simulink model "RR"  (R2024a)
settings: Solver=VariableStepAuto  StartTime=0.0  StopTime=15  RelTol=1e-3  EnableMultiTasking=on
libraries: sm_lib x12, nesl_utility x7
settings Model: Creator=Shashank  LastModifiedBy=ASUS
settings SolverCC: AlgebraicLoopSolver=TrustRegion
settings DataIOCC: LimitDataPoints=on
settings OptimizationCC: LifeSpan=inf
settings DebuggingCC: UnconnectedInputMsg=warning  UnconnectedOutputMsg=warning  UnconnectedLineMsg=warning  AllowSymbolicDim=off  SFUnexpectedBacktrackingDiag=warning  SFNoUnconditionalDefaultTransitionDiag=warning  SFExecutionAtInitializationDiag=none  ArithmeticOperatorsInVariantConditions=warning
settings ModelReferenceCC: EnableRefExpFcnMdlSchedulingChecks=on
settings SFSimCC: SimUseLocalCustomCode=off  CustomCodeUndefinedFunction=UseInterfaceOnly
settings RTWCC: RTWUseLocalCustomCode=off  GPUComputeCapability=3.5
settings CodeAppCC: StateflowObjectComments=on
settings GRTTargetCC: TargetLangStandard=C89/C90 (ANSI)
settings ConfigComp: CovMetricSettings=dw  CovSaveCumulativeToWorkspaceVar=on  CovSaveSingleToWorkspaceVar=on  CovExternalEMLEnable=off  CovSFcnEnable=off
settings SimscapeCC: SimscapeNominalValues="[{\"value\":\"10\",\"unit\":\"V\"},{\"value\":\"1\",\"unit\":\"A\"},{\"value\":\"10\",\"unit\":\"N*m\"},{\"value\":\"10\",\"unit\":\"bar\"},{\"value\":\"100\",\"unit\":\"kJ/kg\"},{\"value\":\"1\",\"unit\":\"kW\"},{\"value\":\"300\",\"unit\":\"K\"},{\"value\":\"100\",\"unit\":\"cm^3/s\"},{\"value\":\"1\",\"unit\":\"kN\"},{\"value\":\"1\",\"unit\":\"g/cm^3\"},{\"value\":\"1\",\"unit\":\"l\"},{\"value\":\"1\",\"unit\":\"cm^2\"},{\"value\":\"60\",\"unit\":\"Hz\"}]"  SimscapeLogType=all  SimscapeLogDataHistory=10000
settings ConfigurationSet: Description=SimMechanics 2G

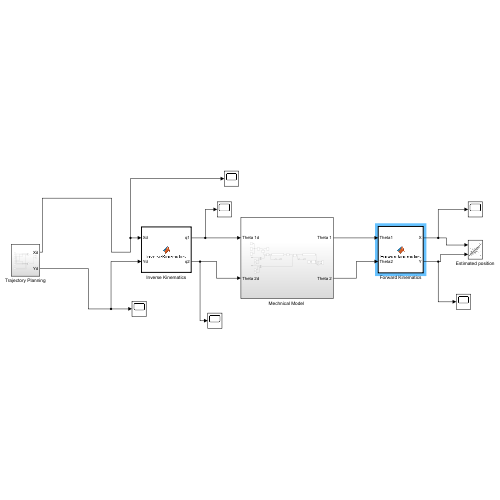
[thumbnail: Simulink's stored preview of the top-level diagram]
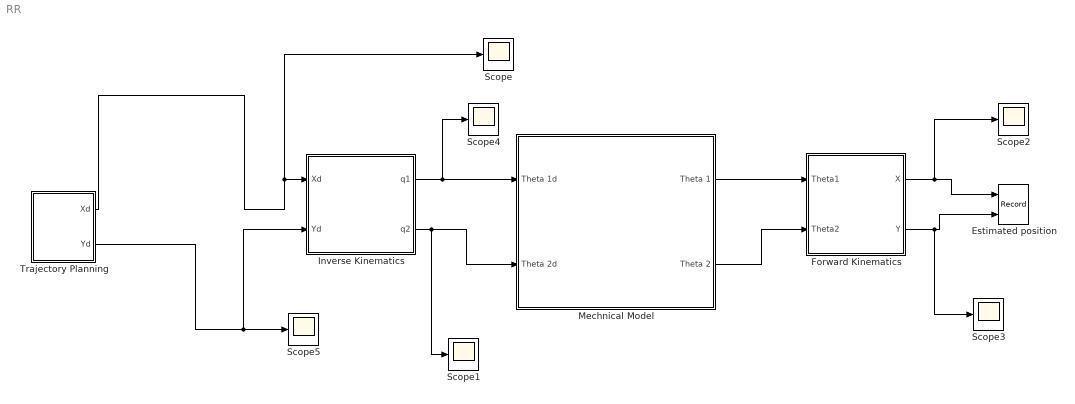
== system RR ==
  Estimated position : Record  FileSettingsInternal="{\"entries\":[{\"content\":{\"excelSettings\":{\"content\":{},\"type\":\"Streamout.ExcelSettings\"}},\"type\":\"Streamout.FileSettingStorage\",\"uuid\":\"\"}],\"packageUris\":[\"http:\\/\\/schema.mathworks.com\\/mf0\\/streamout_blocks\\/R2020a\"],\"version\":\"1.0\"}"  Layout=[1 1]  SignalsInternal="{\"entries\":[{\"content\":{\"signals\":[{\"content\":{\"blockPath\":[],\"dimensions\":[1],\"domain\":\"\",\"lineColor\":\"#a2142f\",\"plots\":[ 1 ],\"port\":1,\"sid\":[\"\"],\"signalID\":1,\"signalName\":\"Forward Kinematics:1\"},\"type\":\"RecordBlkView.Signal\",\"uuid\":\"\"},{\"content\":{\"blockPath\":[],\"dimensions\":[1],\"domain\":\"\",\"lineColor\":\"#139fff\",\"plots\":[ 1 ],\"port\":2,\"sid\":[\"\"],\"signalID\":2,\"signalName\":\"Forward Kinematics:2\"},\"type\":\"RecordBlkView.Signal\",\"uuid\":\"\"}]},\"type\":\"RecordBlkView.InputSignals\",\"uuid\":\"\"}],\"packageUris\":[\"http:\\/\\/schema.mathworks.com\\/mf0\\/streamout_blocks\\/R2020a\"],\"version\":\"1.0\"}"  VisualizationBindings="{\"xyplotplugin\":{\"info\":[{\"series\":[{\"bindingParametersList\":[{\"parameter\":\"X-Axis\",\"signalID\":1,\"signalName\":\"Forward Kinematics:1\"},{\"parameter\":\"Y-Axis\",\"signalID\":2,\"signalName\":\"Forward Kinematics:2\"}],\"seriesID\":0}],\"subplotID\":1}]}}"  CompatibilityTag=XY  st=-1
  Forward Kinematics : MATLAB Function  TreatAsAtomicUnit=on
  Inverse Kinematics : MATLAB Function  TreatAsAtomicUnit=on
  "Mechnical Model " : Subsystem
  Scope{,1..5} (6 alike) : Scope
  Trajectory Planning : Subsystem
  wires:
  Inverse Kinematics/2(q2) -> "Mechnical Model "/2(Theta 2d), Scope1/1
  "Mechnical Model "/1(Theta 1) -> Forward Kinematics/1(Theta1)
  "Mechnical Model "/2(Theta 2) -> Forward Kinematics/2(Theta2)
  Forward Kinematics/1(X) -> Scope2/1, Estimated position/1
  Forward Kinematics/2(Y) -> Scope3/1, Estimated position/2
  Trajectory Planning/1(Xd) -> Inverse Kinematics/1(Xd), Scope/1
  Inverse Kinematics/1(q1) -> Scope4/1, "Mechnical Model "/1(Theta 1d)
  Trajectory Planning/2(Yd) -> Inverse Kinematics/2(Yd), Scope5/1

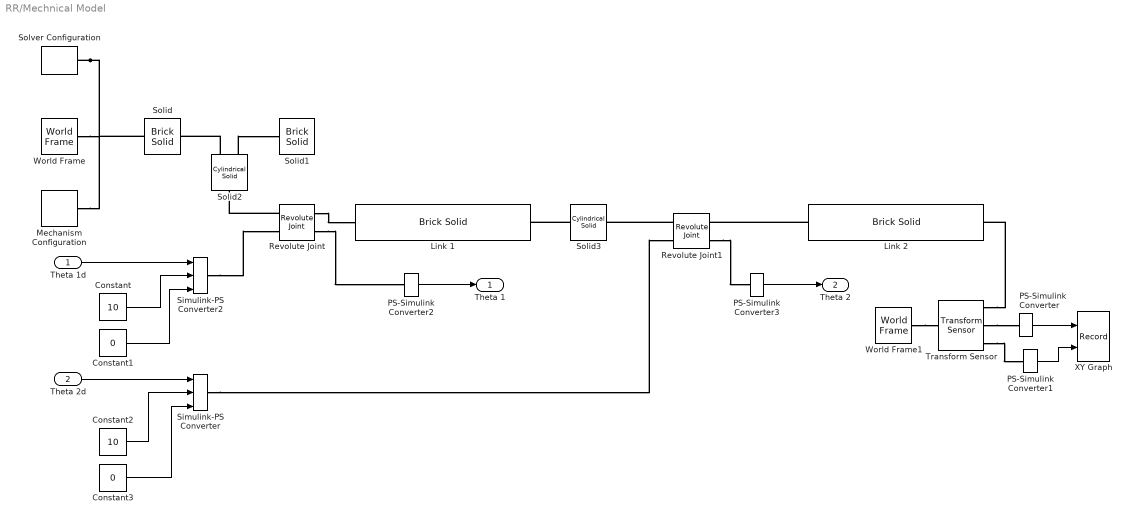
== system RR/Mechnical Model  ==
  Theta 1d : Inport
  Theta 2d : Inport  Port=2
  Constant : Constant  Value=10
  Constant1 : Constant  Value=0
  Constant2 : Constant  Value=10
  Constant3 : Constant  Value=0
  Link 1 : sm_lib/Body Elements/Brick Solid  BrickDimensions=[100 15 5]  BrickDimensionsUnits=cm  ExportEntireGeometry=off  InertiaType=CalculateFromGeometry  BasedOnType=Density  Density=1000  DensityUnits=kg/m^3  Mass=1  MassUnits=kg  CenterOfMass=[0 0 0]  CenterOfMassUnits=m  MomentsOfInertia=[1 1 1]  MomentsOfInertiaUnits=kg*m^2  ProductsOfInertia=[0 0 0]  ProductsOfInertiaUnits=kg*m^2  GraphicType=FromGeometry  MarkerShape=Sphere  MarkerSize=10  GraphicVisPropType=SimpleVisualProperties  GraphicDiffuseColor=[1.0 0.4 0.4]  GraphicOpacity=1.0  GraphicSpecularColor=[0.5 0.5 0.5 1.0]  GraphicAmbientColor=[0.15 0.15 0.15 1.0]  GraphicEmissiveColor=[0.0 0.0 0.0 1.0]  GraphicShininess=75  DoExposeReferenceFrame=off  SerializedFrames=<Frames><Frame><Id>Frame1</Id><Value><Name>L</Name><Origin><Source>GeometricFeature</Source><FeatureName>-x surface</FeatureName></Origin><PrimaryAxis><DefinedDirection>+Z</DefinedDirection><Source>ReferenceFrame</Source><SourceDirection>+Z</SourceDirection><FeatureName></FeatureName></PrimaryAxis><SecondaryAxis><DefinedDirection>+X</DefinedDirection><Source>ReferenceFrame</Source><SourceDirection>+X</SourceDirection><FeatureName></FeatureName></SecondaryAxis></Value></Frame><Frame><Id>Frame2</Id><Value><Name>R</Name><Origin><Source>GeometricFeature</Source><FeatureName>+x surface</FeatureName></Origin><PrimaryAxis><DefinedDirection>+Z</DefinedDirection><Source>ReferenceFrame</Source><SourceDirection>+Z</SourceDirection><FeatureName></FeatureName></PrimaryAxis><SecondaryAxis><DefinedDirection>+X</DefinedDirection><Source>ReferenceFrame</Source><SourceDirection>+X</SourceDirection><FeatureName></FeatureName></SecondaryAxis></Value></Frame></Frames>
  Link 2 : sm_lib/Body Elements/Brick Solid  BrickDimensions=[100 15 5]  BrickDimensionsUnits=cm  ExportEntireGeometry=off  InertiaType=CalculateFromGeometry  BasedOnType=Density  Density=1000  DensityUnits=kg/m^3  Mass=1  MassUnits=kg  CenterOfMass=[0 0 0]  CenterOfMassUnits=m  MomentsOfInertia=[1 1 1]  MomentsOfInertiaUnits=kg*m^2  ProductsOfInertia=[0 0 0]  ProductsOfInertiaUnits=kg*m^2  GraphicType=FromGeometry  MarkerShape=Sphere  MarkerSize=10  GraphicVisPropType=SimpleVisualProperties  GraphicDiffuseColor=[0.0 0.4 0.0]  GraphicOpacity=1.0  GraphicSpecularColor=[0.5 0.5 0.5 1.0]  GraphicAmbientColor=[0.15 0.15 0.15 1.0]  GraphicEmissiveColor=[0.0 0.0 0.0 1.0]  GraphicShininess=75  DoExposeReferenceFrame=off  SerializedFrames=<Frames><Frame><Id>Frame1</Id><Value><Name>L</Name><Origin><Source>GeometricFeature</Source><FeatureName>-x surface</FeatureName></Origin><PrimaryAxis><DefinedDirection>+Z</DefinedDirection><Source>ReferenceFrame</Source><SourceDirection>+Z</SourceDirection><FeatureName></FeatureName></PrimaryAxis><SecondaryAxis><DefinedDirection>+X</DefinedDirection><Source>ReferenceFrame</Source><SourceDirection>+X</SourceDirection><FeatureName></FeatureName></SecondaryAxis></Value></Frame><Frame><Id>Frame2</Id><Value><Name>R</Name><Origin><Source>GeometricFeature</Source><FeatureName>+x surface</FeatureName></Origin><PrimaryAxis><DefinedDirection>+Z</DefinedDirection><Source>ReferenceFrame</Source><SourceDirection>+Z</SourceDirection><FeatureName></FeatureName></PrimaryAxis><SecondaryAxis><DefinedDirection>+X</DefinedDirection><Source>ReferenceFrame</Source><SourceDirection>+X</SourceDirection><FeatureName></FeatureName></SecondaryAxis></Value></Frame></Frames>
  Mechanism Configuration : sm_lib/Utilities/Mechanism Configuration  UniformGravity=Constant  GravityVector=[0 -9.80665 0]  GravityVectorUnits=m/s^2  LinearizationDelta=0.001  JointModeTransitionNonlinearIterations=2
  PS-Simulink Converter{,1..3} (4 alike) : nesl_utility/PS-Simulink Converter  PhysicalDomain=network_engine_domain  SubClassName=ps_output  LeftPortType=input  RightPortType=output  PseudoPeriodic=off  Frequencies=[]  VectorFormat=1-D array  Unit=1  AffineConversion=off
  Revolute Joint : sm_lib/Joints/Revolute Joint  JointMode=Normal  CompositeWrenchDir=FollowerOnBase  CompositeWrenchFrame=BaseFrame  SenseConstraintForce=off  SenseConstraintTorque=off  SenseTotalForce=off  SenseTotalTorque=off  PositionTargetSpecify=off  PositionTargetPriority=High  PositionTargetValue=0  PositionTargetValueUnits=deg  VelocityTargetSpecify=off  VelocityTargetPriority=High  VelocityTargetValue=0  VelocityTargetValueUnits=deg/s  EquilibriumPosition=0  EquilibriumPositionUnits=deg  SpringStiffness=0  SpringStiffnessUnits=N*m/deg  DampingCoefficient=0  DampingCoefficientUnits=N*m/(deg/s)  LowerLimitSpecify=off  LowerLimitBound=-90  LowerLimitBoundUnits=deg  LowerLimitStiffness=1e4  LowerLimitStiffnessUnits=N*m/deg  LowerLimitDamping=10  LowerLimitDampingUnits=N*m/(deg/s)  LowerLimitTransitionRegionWidth=0.1  LowerLimitTransitionRegionWidthUnits=deg  UpperLimitSpecify=off  UpperLimitBound=90  UpperLimitBoundUnits=deg  UpperLimitStiffness=1e4  UpperLimitStiffnessUnits=N*m/deg  UpperLimitDamping=10  UpperLimitDampingUnits=N*m/(deg/s)  UpperLimitTransitionRegionWidth=0.1  UpperLimitTransitionRegionWidthUnits=deg  TorqueActuationMode=ComputedTorque  MotionActuationMode=InputMotion  SensePosition=on  SenseVelocity=off  SenseAcceleration=off  SenseTorqueForce=off  SenseLowerLimitTorqueForce=off  SenseUpperLimitTorqueForce=off
  Revolute Joint1 : sm_lib/Joints/Revolute Joint  JointMode=Normal  CompositeWrenchDir=FollowerOnBase  CompositeWrenchFrame=BaseFrame  SenseConstraintForce=off  SenseConstraintTorque=off  SenseTotalForce=off  SenseTotalTorque=off  PositionTargetSpecify=off  PositionTargetPriority=High  PositionTargetValue=0  PositionTargetValueUnits=deg  VelocityTargetSpecify=off  VelocityTargetPriority=High  VelocityTargetValue=0  VelocityTargetValueUnits=deg/s  EquilibriumPosition=0  EquilibriumPositionUnits=deg  SpringStiffness=0  SpringStiffnessUnits=N*m/deg  DampingCoefficient=0  DampingCoefficientUnits=N*m/(deg/s)  LowerLimitSpecify=off  LowerLimitBound=-90  LowerLimitBoundUnits=deg  LowerLimitStiffness=1e4  LowerLimitStiffnessUnits=N*m/deg  LowerLimitDamping=10  LowerLimitDampingUnits=N*m/(deg/s)  LowerLimitTransitionRegionWidth=0.1  LowerLimitTransitionRegionWidthUnits=deg  UpperLimitSpecify=off  UpperLimitBound=90  UpperLimitBoundUnits=deg  UpperLimitStiffness=1e4  UpperLimitStiffnessUnits=N*m/deg  UpperLimitDamping=10  UpperLimitDampingUnits=N*m/(deg/s)  UpperLimitTransitionRegionWidth=0.1  UpperLimitTransitionRegionWidthUnits=deg  TorqueActuationMode=ComputedTorque  MotionActuationMode=InputMotion  SensePosition=on  SenseVelocity=off  SenseAcceleration=off  SenseTorqueForce=off  SenseLowerLimitTorqueForce=off  SenseUpperLimitTorqueForce=off
  Simulink-PS Converter : nesl_utility/Simulink-PS Converter  PhysicalDomain=network_engine_domain  SubClassName=ps_input  LeftPortType=input  RightPortType=output  PseudoPeriodic=off  Frequencies=[]  NoiseDistribution=none  NoiseParameters=[]  Unit=1  AffineConversion=off  FilteringAndDerivatives=provide  SimscapeFilterOrder=1  InputFilterTimeConstant=0.001  UdotUserProvided=2
  Simulink-PS Converter2 : nesl_utility/Simulink-PS Converter  PhysicalDomain=network_engine_domain  SubClassName=ps_input  LeftPortType=input  RightPortType=output  PseudoPeriodic=off  Frequencies=[]  NoiseDistribution=none  NoiseParameters=[]  Unit=1  AffineConversion=off  FilteringAndDerivatives=provide  SimscapeFilterOrder=1  InputFilterTimeConstant=0.001  UdotUserProvided=2
  Solid : sm_lib/Body Elements/Brick Solid  BrickDimensions=[15 15 5]  BrickDimensionsUnits=cm  ExportEntireGeometry=off  InertiaType=CalculateFromGeometry  BasedOnType=Density  Density=1000  DensityUnits=kg/m^3  Mass=1  MassUnits=kg  CenterOfMass=[0 0 0]  CenterOfMassUnits=m  MomentsOfInertia=[1 1 1]  MomentsOfInertiaUnits=kg*m^2  ProductsOfInertia=[0 0 0]  ProductsOfInertiaUnits=kg*m^2  GraphicType=FromGeometry  MarkerShape=Sphere  MarkerSize=10  GraphicVisPropType=SimpleVisualProperties  GraphicDiffuseColor=[0.0 0.0 0.6]  GraphicOpacity=1.0  GraphicSpecularColor=[0.5 0.5 0.5 1.0]  GraphicAmbientColor=[0.15 0.15 0.15 1.0]  GraphicEmissiveColor=[0.0 0.0 0.0 1.0]  GraphicShininess=75  DoExposeReferenceFrame=on  SerializedFrames=<Frames><Frame><Id>Frame1</Id><Value><Name>F</Name><Origin><Source>GeometricFeature</Source><FeatureName>-z surface</FeatureName></Origin><PrimaryAxis><DefinedDirection>+Z</DefinedDirection><Source>ReferenceFrame</Source><SourceDirection>+Z</SourceDirection><FeatureName></FeatureName></PrimaryAxis><SecondaryAxis><DefinedDirection>+X</DefinedDirection><Source>ReferenceFrame</Source><SourceDirection>+X</SourceDirection><FeatureName></FeatureName></SecondaryAxis></Value></Frame></Frames>
  Solid1 : sm_lib/Body Elements/Brick Solid  BrickDimensions=[15 15 5]  BrickDimensionsUnits=cm  ExportEntireGeometry=off  InertiaType=CalculateFromGeometry  BasedOnType=Density  Density=1000  DensityUnits=kg/m^3  Mass=1  MassUnits=kg  CenterOfMass=[0 0 0]  CenterOfMassUnits=m  MomentsOfInertia=[1 1 1]  MomentsOfInertiaUnits=kg*m^2  ProductsOfInertia=[0 0 0]  ProductsOfInertiaUnits=kg*m^2  GraphicType=FromGeometry  MarkerShape=Sphere  MarkerSize=10  GraphicVisPropType=SimpleVisualProperties  GraphicDiffuseColor=[0.0 0.0 0.6]  GraphicOpacity=1.0  GraphicSpecularColor=[0.5 0.5 0.5 1.0]  GraphicAmbientColor=[0.15 0.15 0.15 1.0]  GraphicEmissiveColor=[0.0 0.0 0.0 1.0]  GraphicShininess=75  DoExposeReferenceFrame=off  SerializedFrames=<Frames><Frame><Id>Frame1</Id><Value><Name>F</Name><Origin><Source>GeometricFeature</Source><FeatureName>+z surface</FeatureName></Origin><PrimaryAxis><DefinedDirection>+Z</DefinedDirection><Source>ReferenceFrame</Source><SourceDirection>+Z</SourceDirection><FeatureName></FeatureName></PrimaryAxis><SecondaryAxis><DefinedDirection>+X</DefinedDirection><Source>ReferenceFrame</Source><SourceDirection>+X</SourceDirection><FeatureName></FeatureName></SecondaryAxis></Value></Frame></Frames>
  Solid2 : sm_lib/Body Elements/Cylindrical Solid  CylinderRadius=5  CylinderRadiusUnits=cm  CylinderLength=6  CylinderLengthUnits=cm  ExportEntireGeometry=off  InertiaType=CalculateFromGeometry  BasedOnType=Density  Density=1000  DensityUnits=kg/m^3  Mass=1  MassUnits=kg  CenterOfMass=[0 0 0]  CenterOfMassUnits=m  MomentsOfInertia=[1 1 1]  MomentsOfInertiaUnits=kg*m^2  ProductsOfInertia=[0 0 0]  ProductsOfInertiaUnits=kg*m^2  GraphicType=FromGeometry  MarkerShape=Sphere  MarkerSize=10  GraphicVisPropType=SimpleVisualProperties  GraphicDiffuseColor=[0.0 0.0 0.6]  GraphicOpacity=1.0  GraphicSpecularColor=[0.5 0.5 0.5 1.0]  GraphicAmbientColor=[0.15 0.15 0.15 1.0]  GraphicEmissiveColor=[0.0 0.0 0.0 1.0]  GraphicShininess=75  DoExposeReferenceFrame=on  SerializedFrames=<Frames><Frame><Id>Frame1</Id><Value><Name>L</Name><Origin><Source>GeometricFeature</Source><FeatureName>top surface</FeatureName></Origin><PrimaryAxis><DefinedDirection>+Z</DefinedDirection><Source>ReferenceFrame</Source><SourceDirection>+Z</SourceDirection><FeatureName></FeatureName></PrimaryAxis><SecondaryAxis><DefinedDirection>+X</DefinedDirection><Source>ReferenceFrame</Source><SourceDirection>+X</SourceDirection><FeatureName></FeatureName></SecondaryAxis></Value></Frame><Frame><Id>Frame2</Id><Value><Name>R</Name><Origin><Source>GeometricFeature</Source><FeatureName>bottom surface</FeatureName></Origin><PrimaryAxis><DefinedDirection>+Z</DefinedDirection><Source>ReferenceFrame</Source><SourceDirection>+Z</SourceDirection><FeatureName></FeatureName></PrimaryAxis><SecondaryAxis><DefinedDirection>+X</DefinedDirection><Source>ReferenceFrame</Source><SourceDirection>+X</SourceDirection><FeatureName></FeatureName></SecondaryAxis></Value></Frame></Frames>
  Solid3 : sm_lib/Body Elements/Cylindrical Solid  CylinderRadius=5  CylinderRadiusUnits=cm  CylinderLength=6  CylinderLengthUnits=cm  ExportEntireGeometry=off  InertiaType=CalculateFromGeometry  BasedOnType=Density  Density=1000  DensityUnits=kg/m^3  Mass=1  MassUnits=kg  CenterOfMass=[0 0 0]  CenterOfMassUnits=m  MomentsOfInertia=[1 1 1]  MomentsOfInertiaUnits=kg*m^2  ProductsOfInertia=[0 0 0]  ProductsOfInertiaUnits=kg*m^2  GraphicType=FromGeometry  MarkerShape=Sphere  MarkerSize=10  GraphicVisPropType=SimpleVisualProperties  GraphicDiffuseColor=[0.8 0.0 0.0]  GraphicOpacity=1.0  GraphicSpecularColor=[0.5 0.5 0.5 1.0]  GraphicAmbientColor=[0.15 0.15 0.15 1.0]  GraphicEmissiveColor=[0.0 0.0 0.0 1.0]  GraphicShininess=75  DoExposeReferenceFrame=off  SerializedFrames=<Frames><Frame><Id>Frame1</Id><Value><Name>L</Name><Origin><Source>GeometricFeature</Source><FeatureName>top surface</FeatureName></Origin><PrimaryAxis><DefinedDirection>+Z</DefinedDirection><Source>ReferenceFrame</Source><SourceDirection>+Z</SourceDirection><FeatureName></FeatureName></PrimaryAxis><SecondaryAxis><DefinedDirection>+X</DefinedDirection><Source>ReferenceFrame</Source><SourceDirection>+X</SourceDirection><FeatureName></FeatureName></SecondaryAxis></Value></Frame><Frame><Id>Frame2</Id><Value><Name>R</Name><Origin><Source>GeometricFeature</Source><FeatureName>bottom surface</FeatureName></Origin><PrimaryAxis><DefinedDirection>+Z</DefinedDirection><Source>ReferenceFrame</Source><SourceDirection>+Z</SourceDirection><FeatureName></FeatureName></PrimaryAxis><SecondaryAxis><DefinedDirection>+X</DefinedDirection><Source>ReferenceFrame</Source><SourceDirection>+X</SourceDirection><FeatureName></FeatureName></SecondaryAxis></Value></Frame></Frames>
  Solver Configuration : nesl_utility/Solver Configuration  PhysicalDomain=network_engine_domain  SubClassName=solver  LeftPortType=input  RightPortType=generic  Tones=[]  Harmonics=[]  SimulateNoise=off  Profile=off  UseLocalSampling=off  EnableSwitchedLinearOptims=on  FrequencyDomain=off  UseCCode=off  RelTol=0.001  AbsTol=1e-06  MinStep=1e-09  ToWorkspace=off  RevertToSquareIcSolve=off  NumHomotopyIterations=100  PhasorMode=off  PhasorModeNumHarmonics=1  ConsistencySolver=NEWTON_FTOL  IndexReductionMethod=DerivativeReplacement  DoDC=off  ResidualTolerance=1e-09  ConsistencyTolSource=GLOBAL  ConsistencyAbsTol=0.001  ConsistencyRelTol=0.001  ConsistencyTolFactor=0.001  UseLocalSolver=off  LocalSolverChoice=NE_BACKWARD_EULER_ADVANCER  ResolveIndetEquations=on  FunctionEvalNumThread=1  LocalSolverSampleTime=0.001  DoFixedCost=off  MaxNonlinIter=3  MaxModeIter=2  ComputeImpulses=off  ImpulseIterations=2  LinearAlgebra=Sparse  LinearAlgebraNumThread=0  EquationFormulation=NE_TIME_EF  DelaysMemoryBudget=1024  AutomaticFiltering=on  FilteringTimeConstant=0.001  PartitionStorageMethod=AS_NEEDED  PartitionMemoryBudget=1024  PartitionMethod=FAST  MultibodyUseLocalSolver=off  MultibodyLocalSolverChoice=ODE1  MultibodyLocalSolverSampleTime=0.001
  Transform Sensor : sm_lib/Frames and Transforms/Transform Sensor  MeasurementFrame=World  RotationSequence=XYX  SenseAngle=off  SenseAxis=off  SenseQ=off  SenseR=off  SenseRotationSequence=off  SenseOmegaX=off  SenseOmegaY=off  SenseOmegaZ=off  SenseOmega=off  SenseQDot=off  SenseRDot=off  SenseRotationSequenceDot=off  SenseAlphaX=off  SenseAlphaY=off  SenseAlphaZ=off  SenseAlpha=off  SenseQDDot=off  SenseRDDot=off  SenseX=on  SenseY=on  SenseZ=off  SenseXYZ=off  SenseRad=off  SenseAzim=off  SenseDist=off  SenseInc=off  SenseXDot=off  SenseYDot=off  SenseZDot=off  SenseXYZDot=off  SenseRadDot=off  SenseAzimDot=off  SenseDistDot=off  SenseIncDot=off  SenseXDDot=off  SenseYDDot=off  SenseZDDot=off  SenseXYZDDot=off  SenseRadDDot=off  SenseAzimDDot=off  SenseDistDDot=off  SenseIncDDot=off
  World Frame : sm_lib/Frames and Transforms/World Frame
  World Frame1 : sm_lib/Frames and Transforms/World Frame
  XY Graph : Record  FileSettingsInternal="{\"entries\":[{\"content\":{\"excelSettings\":{\"content\":{},\"type\":\"Streamout.ExcelSettings\"}},\"type\":\"Streamout.FileSettingStorage\",\"uuid\":\"\"}],\"packageUris\":[\"http:\\/\\/schema.mathworks.com\\/mf0\\/streamout_blocks\\/R2020a\"],\"version\":\"1.0\"}"  Layout=[1 1]  SignalsInternal="{\"entries\":[{\"content\":{\"signals\":[{\"content\":{\"blockPath\":[],\"dimensions\":[1],\"domain\":\"\",\"lineColor\":\"#a2142f\",\"plots\":[ 1 ],\"port\":1,\"sid\":[\"\"],\"signalID\":1,\"signalName\":\"PS-Simulink\\nConverter\"},\"type\":\"RecordBlkView.Signal\",\"uuid\":\"\"},{\"content\":{\"blockPath\":[],\"dimensions\":[1],\"domain\":\"\",\"lineColor\":\"#139fff\",\"plots\":[ 1 ],\"port\":2,\"sid\":[\"\"],\"signalID\":2,\"signalName\":\"PS-Simulink\\nConverter1\"},\"type\":\"RecordBlkView.Signal\",\"uuid\":\"\"}]},\"type\":\"RecordBlkView.InputSignals\",\"uuid\":\"\"}],\"packageUris\":[\"http:\\/\\/schema.mathworks.com\\/mf0\\/streamout_blocks\\/R2020a\"],\"version\":\"1.0\"}"  VisualizationBindings="{\"xyplotplugin\":{\"info\":[{\"series\":[{\"bindingParametersList\":[{\"parameter\":\"X-Axis\",\"signalID\":1,\"signalName\":\"PS-Simulink\\nConverter\"},{\"parameter\":\"Y-Axis\",\"signalID\":2,\"signalName\":\"PS-Simulink\\nConverter1\"}],\"seriesID\":0}],\"subplotID\":1}]}}"  CompatibilityTag=XY  st=-1
  Theta 1 : Outport  VectorParamsAs1DForOutWhenUnconnected=off
  Theta 2 : Outport  Port=2  VectorParamsAs1DForOutWhenUnconnected=off
  wires:
  Constant2/1 -> Simulink-PS Converter/2
  PS-Simulink Converter1/1 -> XY Graph/2
  PS-Simulink Converter/1 -> XY Graph/1
  Constant/1 -> Simulink-PS Converter2/2
  PS-Simulink Converter3/1 -> Theta 2/1
  Theta 2d/1 -> Simulink-PS Converter/1
  PS-Simulink Converter2/1 -> Theta 1/1
  Theta 1d/1 -> Simulink-PS Converter2/1
  Constant1/1 -> Simulink-PS Converter2/3
  Constant3/1 -> Simulink-PS Converter/3
  connections:
  Revolute Joint/RConn2 -- PS-Simulink Converter2/LConn1
  Transform Sensor/RConn1 -- Link 2/RConn1
  Link 2/LConn1 -- Revolute Joint1/RConn1
  Solid2/LConn2 -- Solid1/LConn1
  Revolute Joint/LConn1 -- Solid2/RConn1
  Revolute Joint/RConn1 -- Link 1/LConn1
  Simulink-PS Converter2/RConn1 -- Revolute Joint/LConn2
  Solver Configuration/RConn1 -- Solid/RConn1 -- Mechanism Configuration/RConn1 -- World Frame/RConn1
  Solid3/LConn1 -- Link 1/RConn1
  Transform Sensor/RConn2 -- PS-Simulink Converter/LConn1
  Transform Sensor/RConn3 -- PS-Simulink Converter1/LConn1
  Simulink-PS Converter/RConn1 -- Revolute Joint1/LConn2
  Revolute Joint1/RConn2 -- PS-Simulink Converter3/LConn1
  Solid2/LConn1 -- Solid/LConn1
  World Frame1/RConn1 -- Transform Sensor/LConn1
  Revolute Joint1/LConn1 -- Solid3/RConn1

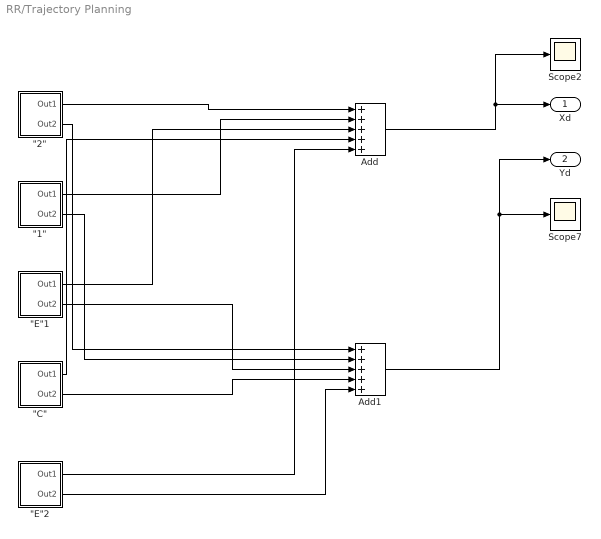
== system RR/Trajectory Planning ==
  "\"1\"" : Subsystem
  "\"2\"" : Subsystem
  "\"C\"" : Subsystem
  "\"E\"1" : Subsystem
  "\"E\"2" : Subsystem
  Add : Sum  Inputs=+++++
  Add1 : Sum  Inputs=+++++
  Scope2 : Scope
  Scope7 : Scope
  Xd : Outport  VectorParamsAs1DForOutWhenUnconnected=off
  Yd : Outport  Port=2  VectorParamsAs1DForOutWhenUnconnected=off
  wires:
  Add/1 -> Scope2/1, Xd/1
  Add1/1 -> Yd/1, Scope7/1
  "\"2\""/1(Out1) -> Add/1
  "\"1\""/1(Out1) -> Add/2
  "\"2\""/2(Out2) -> Add1/1
  "\"1\""/2(Out2) -> Add1/2
  "\"E\"1"/1(Out1) -> Add/3
  "\"E\"1"/2(Out2) -> Add1/3
  "\"C\""/1(Out1) -> Add/4
  "\"C\""/2(Out2) -> Add1/4
  "\"E\"2"/1(Out1) -> Add/5
  "\"E\"2"/2(Out2) -> Add1/5

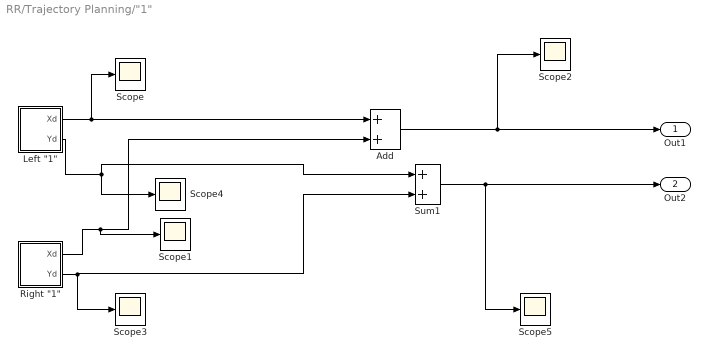
== system RR/Trajectory Planning/"1" ==
  Add : Sum  LockScale=on
  "Left \"1\"" : Subsystem
  "Right \"1\"" : Subsystem
  Scope{,1..5} (6 alike) : Scope
  Sum1 : Sum
  Out1 : Outport
  Out2 : Outport  Port=2
  wires:
  "Left \"1\""/2(Yd) -> Scope4/1, Sum1/1
  "Right \"1\""/2(Yd) -> Scope3/1, Sum1/2
  "Right \"1\""/1(Xd) -> Scope1/1, Add/2
  "Left \"1\""/1(Xd) -> Scope/1, Add/1
  Add/1 -> Scope2/1, Out1/1
  Sum1/1 -> Scope5/1, Out2/1

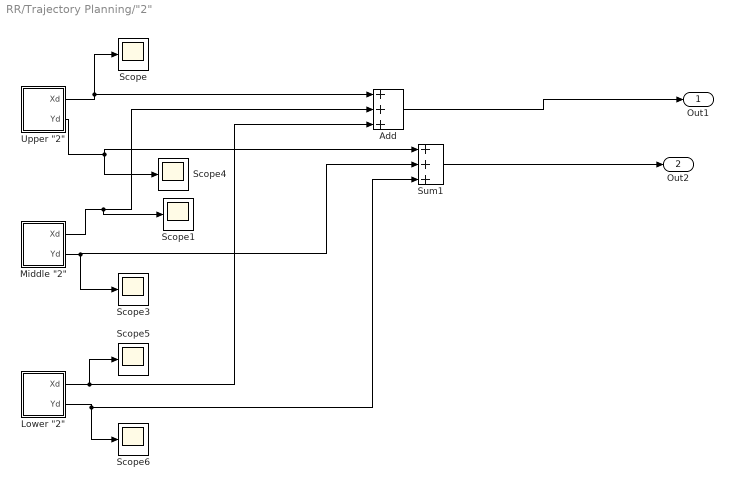
== system RR/Trajectory Planning/"2" ==
  Add : Sum  Inputs=+++  LockScale=on
  "Lower \"2\"" : Subsystem
  "Middle \"2\"" : Subsystem
  Scope{,1,3..6} (6 alike) : Scope
  Sum1 : Sum  Inputs=+++
  "Upper \"2\"" : Subsystem
  Out1 : Outport
  Out2 : Outport  Port=2
  wires:
  "Upper \"2\""/2(Yd) -> Scope4/1, Sum1/1
  "Lower \"2\""/1(Xd) -> Scope5/1, Add/3
  "Middle \"2\""/2(Yd) -> Scope3/1, Sum1/2
  "Middle \"2\""/1(Xd) -> Scope1/1, Add/2
  "Upper \"2\""/1(Xd) -> Scope/1, Add/1
  "Lower \"2\""/2(Yd) -> Sum1/3, Scope6/1
  Add/1 -> Out1/1
  Sum1/1 -> Out2/1

== system RR/Trajectory Planning/"C" ==
  C : Subsystem
  Scope2 : Scope
  Scope5 : Scope
  Out1 : Outport
  Out2 : Outport  Port=2
  wires:
  C/1(Xd) -> Out1/1, Scope2/1
  C/2(Yd) -> Scope5/1, Out2/1

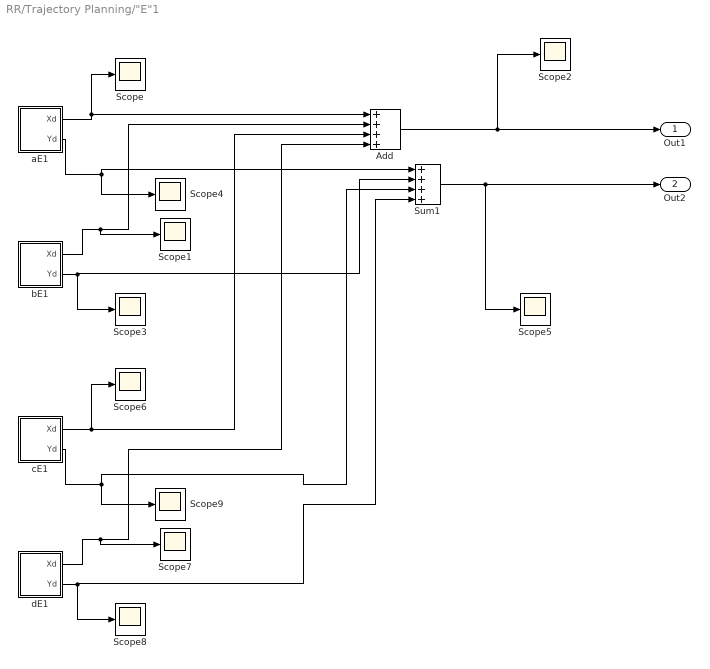
== system RR/Trajectory Planning/"E"1 ==
  Add : Sum  Inputs=++++  LockScale=on
  Scope{,1..9} (10 alike) : Scope
  Sum1 : Sum  Inputs=++++
  aE1 : Subsystem
  bE1 : Subsystem
  cE1 : Subsystem
  dE1 : Subsystem
  Out1 : Outport
  Out2 : Outport  Port=2
  wires:
  aE1/2(Yd) -> Scope4/1, Sum1/1
  bE1/2(Yd) -> Scope3/1, Sum1/2
  bE1/1(Xd) -> Scope1/1, Add/2
  aE1/1(Xd) -> Scope/1, Add/1
  Add/1 -> Scope2/1, Out1/1
  Sum1/1 -> Scope5/1, Out2/1
  cE1/1(Xd) -> Scope6/1, Add/3
  dE1/2(Yd) -> Scope8/1, Sum1/4
  dE1/1(Xd) -> Scope7/1, Add/4
  cE1/2(Yd) -> Scope9/1, Sum1/3

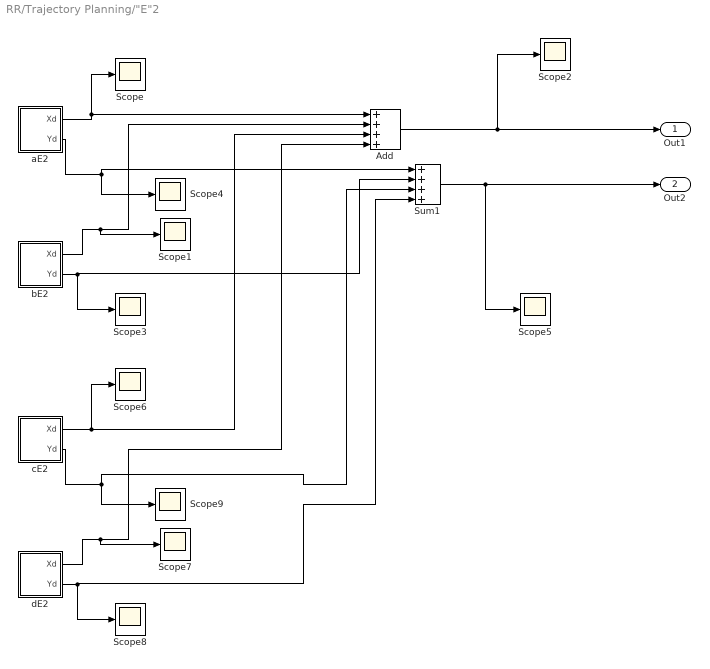
== system RR/Trajectory Planning/"E"2 ==
  Add : Sum  Inputs=++++  LockScale=on
  Scope{,1..9} (10 alike) : Scope
  Sum1 : Sum  Inputs=++++
  aE2 : Subsystem
  bE2 : Subsystem
  cE2 : Subsystem
  dE2 : Subsystem
  Out1 : Outport
  Out2 : Outport  Port=2
  wires:
  aE2/2(Yd) -> Scope4/1, Sum1/1
  bE2/2(Yd) -> Scope3/1, Sum1/2
  bE2/1(Xd) -> Scope1/1, Add/2
  aE2/1(Xd) -> Scope/1, Add/1
  Add/1 -> Scope2/1, Out1/1
  Sum1/1 -> Scope5/1, Out2/1
  cE2/1(Xd) -> Scope6/1, Add/3
  dE2/2(Yd) -> Scope8/1, Sum1/4
  dE2/1(Xd) -> Scope7/1, Add/4
  cE2/2(Yd) -> Scope9/1, Sum1/3

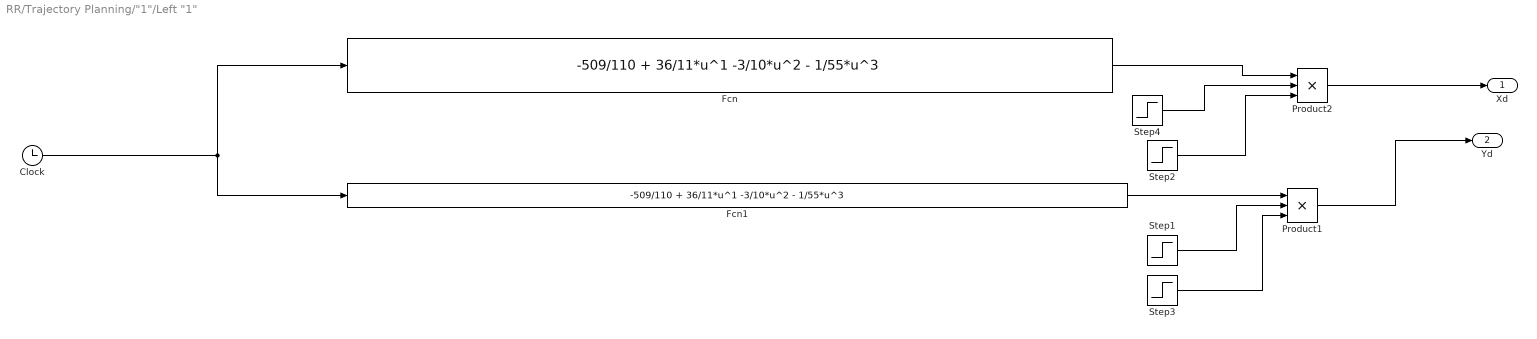
== system RR/Trajectory Planning/"1"/Left "1" ==
  Clock : Clock
  Fcn : Fcn  Expr=-509/110 + 36/11*u^1 -3/10*u^2 - 1/55*u^3
  Fcn1 : Fcn  Expr=-509/110 + 36/11*u^1 -3/10*u^2 - 1/55*u^3
  Product1 : Product  Inputs=3
  Product2 : Product  Inputs=3
  Step1 : Step  Time=3  SampleTime=0
  Step2 : Step  Time=4  Before=1  After=0  SampleTime=0
  Step3 : Step  Time=4  Before=1  After=0  SampleTime=0
  Step4 : Step  Time=3  SampleTime=0
  Xd : Outport
  Yd : Outport  Port=2
  wires:
  Clock/1 -> Fcn1/1, Fcn/1
  Fcn/1 -> Product2/1
  Product2/1 -> Xd/1
  Fcn1/1 -> Product1/1
  Product1/1 -> Yd/1
  Step4/1 -> Product2/2
  Step2/1 -> Product2/3
  Step1/1 -> Product1/2
  Step3/1 -> Product1/3

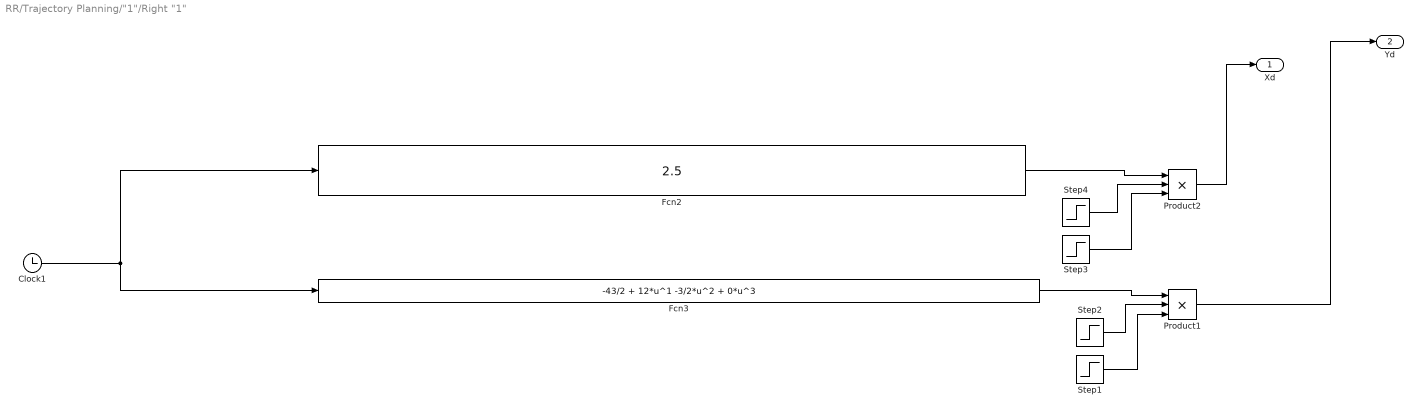
== system RR/Trajectory Planning/"1"/Right "1" ==
  Clock1 : Clock
  Fcn2 : Fcn  Expr=2.5
  Fcn3 : Fcn  Expr=-43/2 + 12*u^1 -3/2*u^2 + 0*u^3
  Product1 : Product  Inputs=3
  Product2 : Product  Inputs=3
  Step1 : Step  Time=5  Before=1  After=0  SampleTime=0
  Step2 : Step  Time=4  SampleTime=0
  Step3 : Step  Time=5  Before=1  After=0  SampleTime=0
  Step4 : Step  Time=4  SampleTime=0
  Xd : Outport
  Yd : Outport  Port=2
  wires:
  Product1/1 -> Yd/1
  Fcn2/1 -> Product2/1
  Step3/1 -> Product2/3
  Clock1/1 -> Fcn2/1, Fcn3/1
  Step1/1 -> Product1/3
  Step4/1 -> Product2/2
  Fcn3/1 -> Product1/1
  Step2/1 -> Product1/2
  Product2/1 -> Xd/1

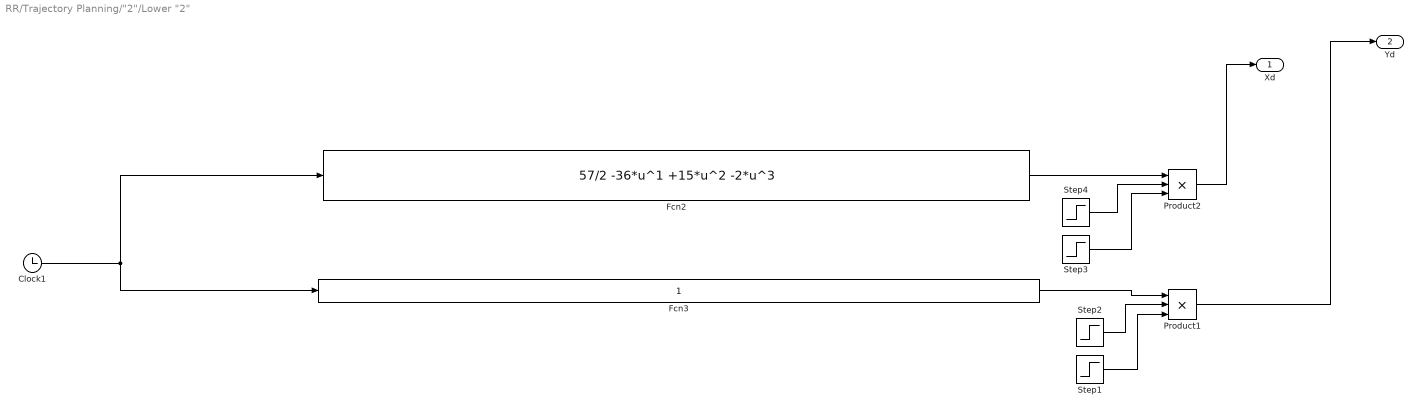
== system RR/Trajectory Planning/"2"/Lower "2" ==
  Clock1 : Clock
  Fcn2 : Fcn  Expr=57/2 -36*u^1 +15*u^2 -2*u^3
  Fcn3 : Fcn  Expr=1
  Product1 : Product  Inputs=3
  Product2 : Product  Inputs=3
  Step1 : Step  Time=3  Before=1  After=0  SampleTime=0
  Step2 : Step  Time=2  SampleTime=0
  Step3 : Step  Time=3  Before=1  After=0  SampleTime=0
  Step4 : Step  Time=2  SampleTime=0
  Xd : Outport
  Yd : Outport  Port=2
  wires:
  Product1/1 -> Yd/1
  Fcn2/1 -> Product2/1
  Step3/1 -> Product2/3
  Clock1/1 -> Fcn2/1, Fcn3/1
  Step1/1 -> Product1/3
  Step4/1 -> Product2/2
  Fcn3/1 -> Product1/1
  Step2/1 -> Product1/2
  Product2/1 -> Xd/1

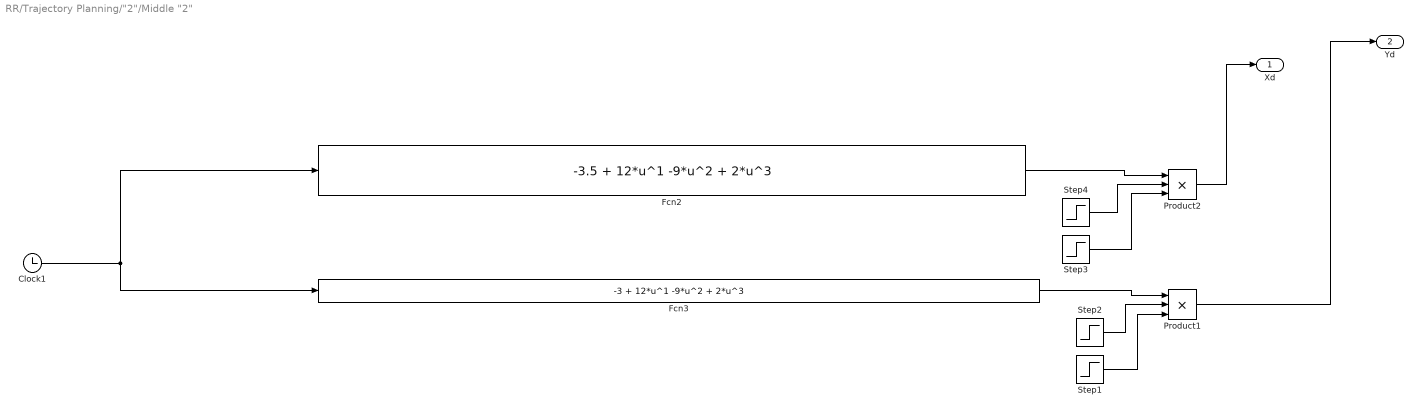
== system RR/Trajectory Planning/"2"/Middle "2" ==
  Clock1 : Clock
  Fcn2 : Fcn  Expr=-3.5 + 12*u^1 -9*u^2 + 2*u^3
  Fcn3 : Fcn  Expr=-3 + 12*u^1 -9*u^2 + 2*u^3
  Product1 : Product  Inputs=3
  Product2 : Product  Inputs=3
  Step1 : Step  Time=2  Before=1  After=0  SampleTime=0
  Step2 : Step  Time=1.000000000000000000000000000001  SampleTime=0
  Step3 : Step  Time=2  Before=1  After=0  SampleTime=0
  Step4 : Step  Time=1.00000000000000000000000001  SampleTime=0
  Xd : Outport
  Yd : Outport  Port=2
  wires:
  Product1/1 -> Yd/1
  Fcn2/1 -> Product2/1
  Step3/1 -> Product2/3
  Clock1/1 -> Fcn2/1, Fcn3/1
  Step1/1 -> Product1/3
  Step4/1 -> Product2/2
  Fcn3/1 -> Product1/1
  Step2/1 -> Product1/2
  Product2/1 -> Xd/1

== system RR/Trajectory Planning/"2"/Upper "2" ==
  Clock : Clock
  Fcn : Fcn  Expr=0.5 + 0*u^1 + 3*u^2 - 2*u^3
  Fcn1 : Fcn  Expr=2 + 0.5*sin((pi)*(u-1)-pi)
  Product1 : Product
  Product2 : Product
  Step1 : Step  Before=1  After=0  SampleTime=0
  Step3 : Step  Before=1  After=0  SampleTime=0
  Xd : Outport
  Yd : Outport  Port=2
  wires:
  Clock/1 -> Fcn1/1, Fcn/1
  Fcn/1 -> Product2/1
  Product2/1 -> Xd/1
  Step3/1 -> Product2/2
  Fcn1/1 -> Product1/1
  Step1/1 -> Product1/2
  Product1/1 -> Yd/1

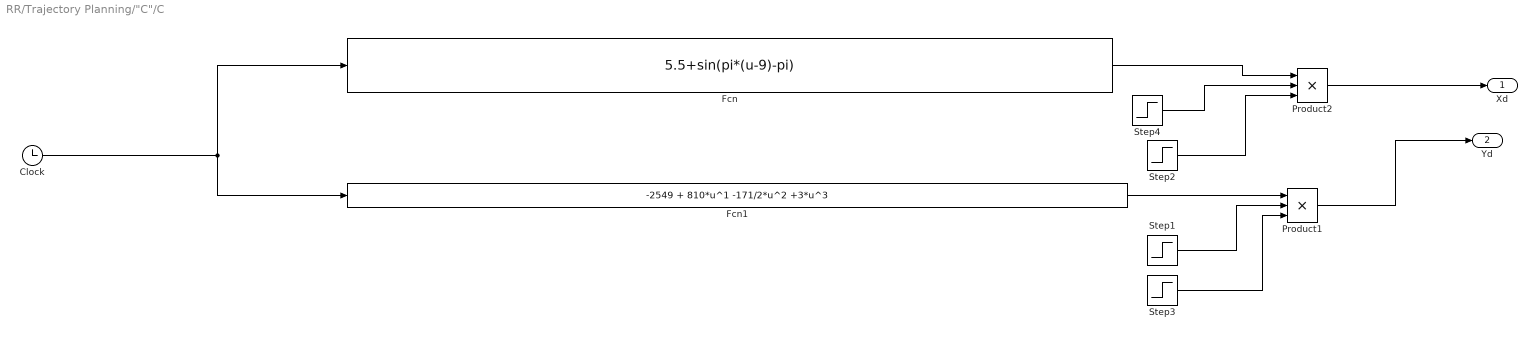
== system RR/Trajectory Planning/"C"/C ==
  Clock : Clock
  Fcn : Fcn  Expr=5.5+sin(pi*(u-9)-pi)
  Fcn1 : Fcn  Expr=-2549 + 810*u^1 -171/2*u^2 +3*u^3
  Product1 : Product  Inputs=3
  Product2 : Product  Inputs=3
  Step1 : Step  Time=9  SampleTime=0
  Step2 : Step  Time=10  Before=1  After=0  SampleTime=0
  Step3 : Step  Time=10  Before=1  After=0  SampleTime=0
  Step4 : Step  Time=9  SampleTime=0
  Xd : Outport
  Yd : Outport  Port=2
  wires:
  Clock/1 -> Fcn1/1, Fcn/1
  Fcn/1 -> Product2/1
  Product2/1 -> Xd/1
  Fcn1/1 -> Product1/1
  Product1/1 -> Yd/1
  Step4/1 -> Product2/2
  Step2/1 -> Product2/3
  Step1/1 -> Product1/2
  Step3/1 -> Product1/3

== system RR/Trajectory Planning/"E"1/aE1 ==
  Clock : Clock
  Fcn : Fcn  Expr=3
  Fcn1 : Fcn  Expr=-485 + 270*u^1 -99/2*u^2 +3*u^3
  Product1 : Product  Inputs=3
  Product2 : Product  Inputs=3
  Step1 : Step  Time=5  SampleTime=0
  Step2 : Step  Time=6  Before=1  After=0  SampleTime=0
  Step3 : Step  Time=6  Before=1  After=0  SampleTime=0
  Step4 : Step  Time=5  SampleTime=0
  Xd : Outport
  Yd : Outport  Port=2
  wires:
  Clock/1 -> Fcn1/1, Fcn/1
  Fcn/1 -> Product2/1
  Product2/1 -> Xd/1
  Fcn1/1 -> Product1/1
  Product1/1 -> Yd/1
  Step4/1 -> Product2/2
  Step2/1 -> Product2/3
  Step1/1 -> Product1/2
  Step3/1 -> Product1/3

== system RR/Trajectory Planning/"E"1/bE1 ==
  Clock1 : Clock
  Fcn2 : Fcn  Expr=543 -252*u^1 +39*u^2 -2*u^3
  Fcn3 : Fcn  Expr=2.5
  Product1 : Product  Inputs=3
  Product2 : Product  Inputs=3
  Step1 : Step  Time=7  Before=1  After=0  SampleTime=0
  Step2 : Step  Time=6  SampleTime=0
  Step3 : Step  Time=7  Before=1  After=0  SampleTime=0
  Step4 : Step  Time=6  SampleTime=0
  Xd : Outport
  Yd : Outport  Port=2
  wires:
  Product1/1 -> Yd/1
  Fcn2/1 -> Product2/1
  Step3/1 -> Product2/3
  Clock1/1 -> Fcn2/1, Fcn3/1
  Step1/1 -> Product1/3
  Step4/1 -> Product2/2
  Fcn3/1 -> Product1/1
  Step2/1 -> Product1/2
  Product2/1 -> Xd/1

== system RR/Trajectory Planning/"E"1/cE1 ==
  Clock : Clock
  Fcn : Fcn  Expr=836 - 336*u^1 +45*u^2 - 2*u^3
  Fcn1 : Fcn  Expr=1.75
  Product1 : Product  Inputs=3
  Product2 : Product  Inputs=3
  Step1 : Step  Time=7  SampleTime=0
  Step2 : Step  Time=8  Before=1  After=0  SampleTime=0
  Step3 : Step  Time=8  Before=1  After=0  SampleTime=0
  Step4 : Step  Time=7  SampleTime=0
  Xd : Outport
  Yd : Outport  Port=2
  wires:
  Clock/1 -> Fcn1/1, Fcn/1
  Fcn/1 -> Product2/1
  Product2/1 -> Xd/1
  Fcn1/1 -> Product1/1
  Product1/1 -> Yd/1
  Step4/1 -> Product2/2
  Step2/1 -> Product2/3
  Step1/1 -> Product1/2
  Step3/1 -> Product1/3

== system RR/Trajectory Planning/"E"1/dE1 ==
  Clock1 : Clock
  Fcn2 : Fcn  Expr=1219 -432*u^1 +51*u^2 -2*u^3
  Fcn3 : Fcn  Expr=1
  Product1 : Product  Inputs=3
  Product2 : Product  Inputs=3
  Step1 : Step  Time=9  Before=1  After=0  SampleTime=0
  Step2 : Step  Time=8  SampleTime=0
  Step3 : Step  Time=9  Before=1  After=0  SampleTime=0
  Step4 : Step  Time=8  SampleTime=0
  Xd : Outport
  Yd : Outport  Port=2
  wires:
  Product1/1 -> Yd/1
  Fcn2/1 -> Product2/1
  Step3/1 -> Product2/3
  Clock1/1 -> Fcn2/1, Fcn3/1
  Step1/1 -> Product1/3
  Step4/1 -> Product2/2
  Fcn3/1 -> Product1/1
  Step2/1 -> Product1/2
  Product2/1 -> Xd/1

== system RR/Trajectory Planning/"E"2/aE2 ==
  Clock : Clock
  Fcn : Fcn  Expr=6
  Fcn1 : Fcn  Expr=-6895/2 + 990*u^1 -189/2*u^2 +3*u^3
  Product1 : Product  Inputs=3
  Product2 : Product  Inputs=3
  Step1 : Step  Time=10  SampleTime=0
  Step2 : Step  Time=11  Before=1  After=0  SampleTime=0
  Step3 : Step  Time=11  Before=1  After=0  SampleTime=0
  Step4 : Step  Time=10  SampleTime=0
  Xd : Outport
  Yd : Outport  Port=2
  wires:
  Clock/1 -> Fcn1/1, Fcn/1
  Fcn/1 -> Product2/1
  Product2/1 -> Xd/1
  Fcn1/1 -> Product1/1
  Product1/1 -> Yd/1
  Step4/1 -> Product2/2
  Step2/1 -> Product2/3
  Step1/1 -> Product1/2
  Step3/1 -> Product1/3

== system RR/Trajectory Planning/"E"2/bE2 ==
  Clock1 : Clock
  Fcn2 : Fcn  Expr=3031 -792*u^1 +69*u^2 -2*u^3
  Fcn3 : Fcn  Expr=2.5
  Product1 : Product  Inputs=3
  Product2 : Product  Inputs=3
  Step1 : Step  Time=12  Before=1  After=0  SampleTime=0
  Step2 : Step  Time=11  SampleTime=0
  Step3 : Step  Time=12  Before=1  After=0  SampleTime=0
  Step4 : Step  Time=11  SampleTime=0
  Xd : Outport
  Yd : Outport  Port=2
  wires:
  Product1/1 -> Yd/1
  Fcn2/1 -> Product2/1
  Step3/1 -> Product2/3
  Clock1/1 -> Fcn2/1, Fcn3/1
  Step1/1 -> Product1/3
  Step4/1 -> Product2/2
  Fcn3/1 -> Product1/1
  Step2/1 -> Product1/2
  Product2/1 -> Xd/1

== system RR/Trajectory Planning/"E"2/cE2 ==
  Clock : Clock
  Fcn : Fcn  Expr=3894 -936*u^1 +75*u^2 -2*u^3
  Fcn1 : Fcn  Expr=1.75
  Product1 : Product  Inputs=3
  Product2 : Product  Inputs=3
  Step1 : Step  Time=12  SampleTime=0
  Step2 : Step  Time=13  Before=1  After=0  SampleTime=0
  Step3 : Step  Time=13  Before=1  After=0  SampleTime=0
  Step4 : Step  Time=12  SampleTime=0
  Xd : Outport
  Yd : Outport  Port=2
  wires:
  Clock/1 -> Fcn1/1, Fcn/1
  Fcn/1 -> Product2/1
  Product2/1 -> Xd/1
  Fcn1/1 -> Product1/1
  Product1/1 -> Yd/1
  Step4/1 -> Product2/2
  Step2/1 -> Product2/3
  Step1/1 -> Product1/2
  Step3/1 -> Product1/3

== system RR/Trajectory Planning/"E"2/dE2 ==
  Clock1 : Clock
  Fcn2 : Fcn  Expr=4907 -1092*u^1 +81*u^2 -2*u^3
  Fcn3 : Fcn  Expr=1
  Product1 : Product  Inputs=3
  Product2 : Product  Inputs=3
  Step1 : Step  Time=14  Before=1  After=0  SampleTime=0
  Step2 : Step  Time=13  SampleTime=0
  Step3 : Step  Time=14  Before=1  After=0  SampleTime=0
  Step4 : Step  Time=13  SampleTime=0
  Xd : Outport
  Yd : Outport  Port=2
  wires:
  Product1/1 -> Yd/1
  Fcn2/1 -> Product2/1
  Step3/1 -> Product2/3
  Clock1/1 -> Fcn2/1, Fcn3/1
  Step1/1 -> Product1/3
  Step4/1 -> Product2/2
  Fcn3/1 -> Product1/1
  Step2/1 -> Product1/2
  Product2/1 -> Xd/1

== matlab function RR/Inverse Kinematics ==
  data: q1 output; q2 output; Xd input; Yd input
function [q1,q2] = InverseKinematics(Xd,Yd)

l1 = 4;
l2 = 4;

q2 = -real(acos(complex((Xd^2+Yd^2 - l1^2 - l2^2)/(2*l1*l2))));

s_q2 = sin(q2);
c_q2 = cos(q2);

q1 = atan2(Yd,Xd) - atan2(real(l2*s_q2), real((l1+l2*c_q2)));

== matlab function RR/Forward Kinematics ==
  data: Theta1 input; X output; Theta2 input; Y output
function [X,Y] = Forwardkinematics(Theta1, Theta2)

l1 =4;
l2 = 4;

T10 = [cos(Theta1), -sin(Theta1), 0, l1*cos(Theta1);
    sin(Theta1), cos(Theta1), 0, l1*sin(Theta1);
    0, 0, 1, 0;
    0, 0, 0, 1];

T21 = [cos(Theta2), -sin(Theta2), 0, l1*cos(Theta2);
    sin(Theta2), cos(Theta2), 0, l1*sin(Theta2);
    0, 0, 1, 0;
    0, 0, 0, 1];

T20 = T10*T21;

X = T20(1,4);
Y = T20(2,4);
